simulink model "SimulacionClase3"  (R2022a)
settings: Solver=VariableStepAuto  StartTime=0.0  StopTime=100.0  RelTol=1e-3
values from neighbouring files (symbols this model uses):
  A = [1 -1 0.01 0.12]    [Real_Esta_Disc_Ref.m]    (also in Routh_Hurwitz.m = [0 1 0;0 0 1;-160 -56 -14]; Smulacro_Parcial_Final.m = matrizA; observador_estados_ex1.m = [-20 1 ;-1 0]; tercer_orden.m = 1)
  B = 0.00223579    [CompensadordicretoVelocidadLGR.m]    (also in Real_Esta_Disc_Ref.m = [0 0 1 0.5]; Routh_Hurwitz.m = [0;1;-14]; Smulacro_Parcial_Final.m = matrizB; tercer_orden.m = -0.947368468698)
  C = tf(Kc*[ti*td ti 1],[ti 0])    [PID_Ku.m]    (also in Raices.m = (s^2+2*zeta*wn*s+wn^2)/(0.1*s+1); Routh_Hurwitz.m = [1 0 0]; Smulacro_Parcial_Final.m = matrizC; diseñoCompensadorAdelanto.m = leadlag(K, Td, Ti))
  ki = -50.9664    [Control.m]
undefined symbols (not defined in the file or in its folder): K12, ke
libraries: simulink x1
settings Model: Creator=Juan  LastModifiedBy=Juan

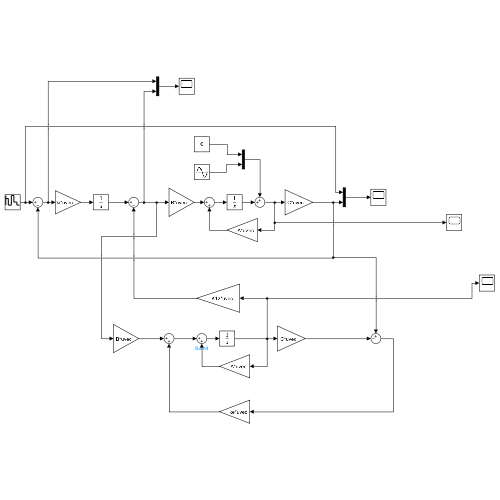
[thumbnail: Simulink's stored preview of the top-level diagram]
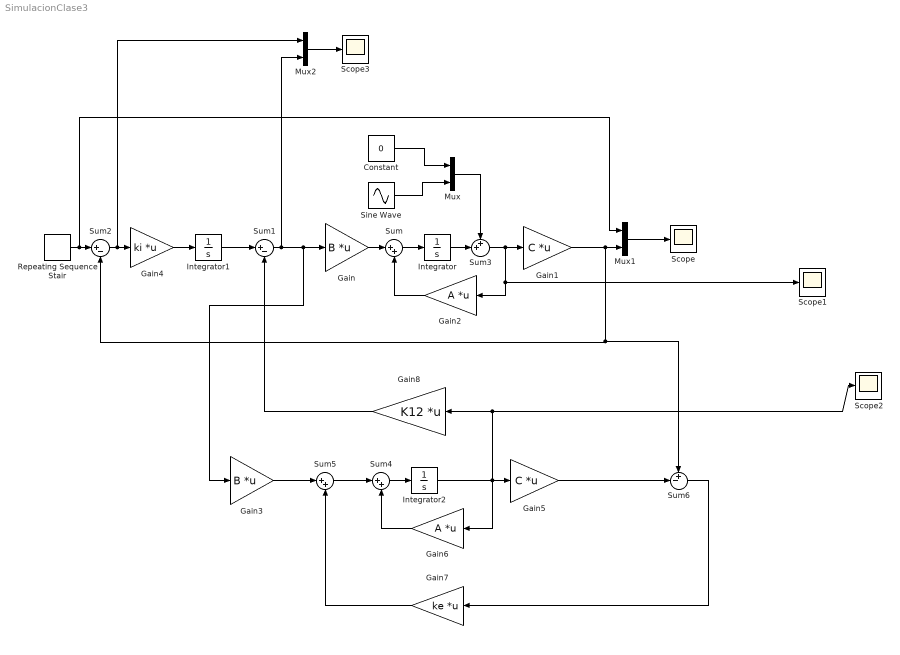
== system SimulacionClase3 ==
  Constant : Constant  Value=0
  Gain : Gain  Gain=B  Multiplication=Matrix(K*u) (u vector)
  Gain1 : Gain  Gain=C  Multiplication=Matrix(K*u) (u vector)
  Gain2 : Gain  Gain=A  Multiplication=Matrix(K*u) (u vector)
  Gain3 : Gain  Gain=B  Multiplication=Matrix(K*u) (u vector)
  Gain4 : Gain  Gain=ki  Multiplication=Matrix(K*u) (u vector)
  Gain5 : Gain  Gain=C  Multiplication=Matrix(K*u) (u vector)
  Gain6 : Gain  Gain=A  Multiplication=Matrix(K*u) (u vector)
  Gain7 : Gain  Gain=ke  Multiplication=Matrix(K*u) (u vector)
  Gain8 : Gain  Gain=K12  Multiplication=Matrix(K*u) (u vector)
  Integrator : Integrator
  Integrator1 : Integrator
  Integrator2 : Integrator
  Mux : Mux  Inputs=2
  Mux1 : Mux  Inputs=2
  Mux2 : Mux  Inputs=2
  Repeating Sequence Stair : simulink/Sources/Repeating Sequence Stair  OutValues=[3 1 4 2 1].'  tsamp=20  OutMin=[]  OutMax=[]  OutDataTypeStr=double  OutputDataTypeScalingMode=double  OutDataType=fixdt(0,8)  ConRadixGroup=Best Precision: Vector-wise  OutScaling=2^-12
  Scope{,1..3} (4 alike) : Scope
  Sine Wave : Sin  Amplitude=0.01  Frequency=100  SampleTime=0
  Sum : Sum  Inputs=|++
  Sum1 : Sum  Inputs=|+-
  Sum2 : Sum  Inputs=|+-
  Sum3 : Sum  Inputs=++|
  Sum4 : Sum  Inputs=|++
  Sum5 : Sum  Inputs=|++
  Sum6 : Sum  Inputs=+-|
  wires:
  Integrator1/1 -> Sum1/1
  Sum/1 -> Integrator/1
  Mux1/1 -> Scope/1
  Gain1/1 -> Mux1/2, Sum6/1, Sum2/2
  Gain2/1 -> Sum/2
  Repeating Sequence Stair/1 -> Mux1/1, Sum2/1
  Gain/1 -> Sum/1
  Sine Wave/1 -> Mux/2
  Integrator/1 -> Sum3/2
  Constant/1 -> Mux/1
  Sum3/1 -> Scope1/1, Gain2/1, Gain1/1
  Gain4/1 -> Integrator1/1
  Mux/1 -> Sum3/1
  Sum4/1 -> Integrator2/1
  Gain6/1 -> Sum4/2
  Integrator2/1 -> Scope2/1, Gain8/1, Gain6/1, Gain5/1
  Sum5/1 -> Sum4/1
  Gain3/1 -> Sum5/1
  Gain7/1 -> Sum5/2
  Gain5/1 -> Sum6/2
  Sum6/1 -> Gain7/1
  Gain8/1 -> Sum1/2
  Sum1/1 -> Mux2/2, Gain3/1, Gain/1
  Sum2/1 -> Mux2/1, Gain4/1
  Mux2/1 -> Scope3/1
